simulink model "Biomasa_modelling"  (R2018a)
settings: Solver=ode23  StartTime=0.0  StopTime=120  RelTol=1e-3
InitFcn:
  | parametros_BIO
values from neighbouring files (symbols this model uses):
  b = 4.91    [SimulinkInit.m]    (also in parametros_BIO.m)
  C = 1    [SimulinkInit.m]    (also in parametros_BIO.m)
  K = 25    [SimulinkInit.m]    (also in parametros_BIO.m; uio_linear.m = K1+E*H)
  K1 = 9.66    [SimulinkInit.m]    (also in parametros_BIO.m; uio_linear.m = K1')
  K11 = 0.8    [SimulinkInit.m]    (also in parametros_BIO.m)
  K2 = 6.97    [SimulinkInit.m]    (also in parametros_BIO.m)
  K22 = 0.2    [SimulinkInit.m]    (also in parametros_BIO.m)
  K3 = 31.8    [SimulinkInit.m]    (also in parametros_BIO.m)
  K33 = 0.23    [SimulinkInit.m]    (also in parametros_BIO.m)
  K4 = 15.1    [SimulinkInit.m]    (also in parametros_BIO.m)
  Kd = 0.02    [SimulinkInit.m]    (also in parametros_BIO.m)
  Kdc = 0.02    [SimulinkInit.m]    (also in parametros_BIO.m)
  Kf = 1    [SimulinkInit.m]    (also in parametros_BIO.m)
  Kh = 1.2    [SimulinkInit.m]    (also in parametros_BIO.m)
  Ks = 21.5    [SimulinkInit.m]    (also in parametros_BIO.m)
  Ksc = 3    [SimulinkInit.m]    (also in parametros_BIO.m)
  Kv = 1    [SimulinkInit.m]    (also in parametros_BIO.m)
  Sbin = 13.8    [SimulinkInit.m]    (also in parametros_BIO.m)
  Svin = 2.91    [SimulinkInit.m]    (also in parametros_BIO.m)
  T1 = 0.4    [SimulinkInit.m]    (also in parametros_BIO.m)
  T2 = 1    [SimulinkInit.m]    (also in parametros_BIO.m)
  T3 = 15    [SimulinkInit.m]    (also in parametros_BIO.m)
  T4 = 2.5    [SimulinkInit.m]    (also in parametros_BIO.m)
  T5 = 3.3    [SimulinkInit.m]    (also in parametros_BIO.m)
  Tcd = 0.2    [SimulinkInit.m]    (also in parametros_BIO.m)
  Tcr = 0.01    [SimulinkInit.m]    (also in parametros_BIO.m)
  Tf = 0.04    [SimulinkInit.m]    (also in parametros_BIO.m)
  Tr = 950    [SimulinkInit.m]    (also in parametros_BIO.m)
  Tt = 450    [SimulinkInit.m]    (also in parametros_BIO.m)
  Ttd = 0.04    [SimulinkInit.m]    (also in parametros_BIO.m)
  Tv = 0.05    [SimulinkInit.m]    (also in parametros_BIO.m)
  V = 20    [SimulinkInit.m]    (also in parametros_BIO.m)
  wref = 70000    [SimulinkInit.m]    (also in parametros_BIO.m)
  X_acid = 1.2    [SimulinkInit.m]    (also in parametros_BIO.m)
  X_meth = 0.35    [SimulinkInit.m]    (also in parametros_BIO.m)
  Z = 3    [SimulinkInit.m]    (also in parametros_BIO.m)
libraries: powerlib x3
settings Model: Creator=cmparedes  LastModifiedBy=cmparedes
settings SolverCC: AlgebraicLoopSolver=LineSearch

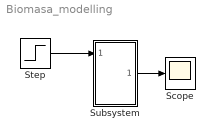
== system Biomasa_modelling ==
  Scope : Scope
  Step : Step  Time=0  After=28  SampleTime=0
  Subsystem : Subsystem
  wires:
  Step/1 -> Subsystem/1(In1)
  Subsystem/1(Vdc) -> Scope/1

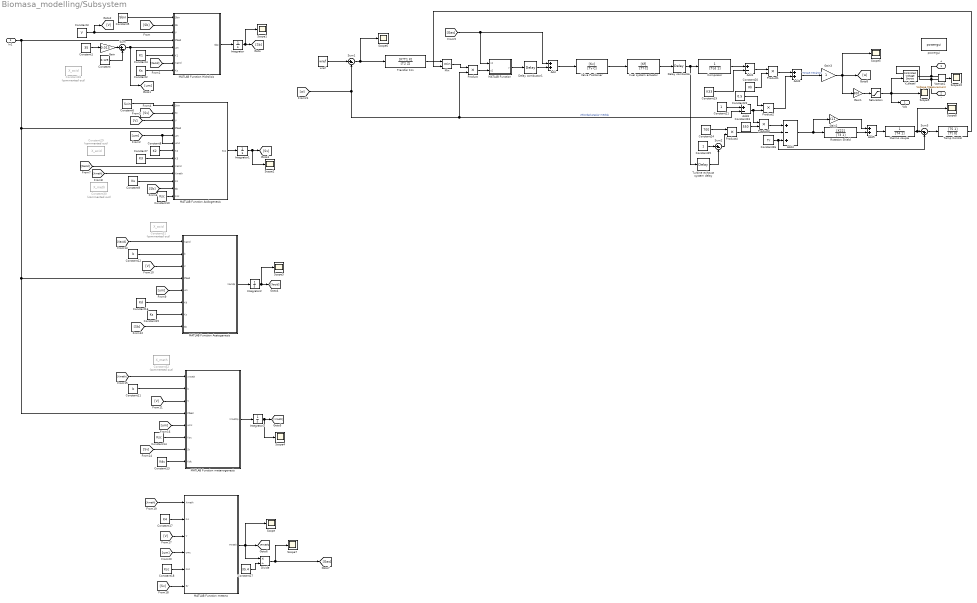
== system Biomasa_modelling/Subsystem ==
  In1 : Inport
  Add : Sum
  Add1 : Sum  Inputs=+-
  Add2 : Sum
  Add3 : Sum  Inputs=+-
  Add4 : Sum  Inputs=+-+
  Add5 : Sum
  Compresor : TransferFcn  Denominator=[Tcd 1]
  Constant : Constant  Value=0.129
  Constant1 : Constant  Value=35
  Constant10 : Constant  Value=Ksc
  Constant11 : Constant  Value=b
  Constant12 : Constant  Value=b
  Constant13 : Constant  Value=Kdc
  Constant14 : Constant  Value=Ksc
  Constant15 : Constant  Value=Ks
  Constant16 : Constant  Value=Kd
  Constant17 : Constant  Value=K4
  Constant18 : Constant  Value=Ksc
  Constant19 : Constant  Value=K33
  Constant2 : Constant  Value=Ks
  Constant20 : Constant  Value=Kh
  Constant21 : Constant
  Constant22 : Constant  Value=0.5
  Constant23 : Constant  Value=550
  Constant24 : Constant  Value=700
  Constant25 : Constant
  Constant26 : Constant  Value=Tr
  Constant27 : Constant  Value=35.4
  Constant28 : Constant  Commented=on  Value=X_acid
  Constant29 : Constant  Commented=on  Value=X_acid
  Constant3 : Constant  Value=V
  Constant30 : Constant  Commented=on  Value=X_meth
  Constant31 : Constant  Commented=on  Value=X_acid
  Constant32 : Constant  Commented=on  Value=X_meth
  Constant4 : Constant  Value=K1
  Constant5 : Constant  Value=Sbin
  Constant6 : Constant  Value=Svin
  Constant7 : Constant  Value=K3
  Constant8 : Constant  Value=K2
  Constant9 : Constant  Value=Ks
  Delay combustor : TransportDelay  DelayTime=Tcr
  Delay combustor1 : TransportDelay  DelayTime=0
  Divide : Product  Inputs=*/
  Fuel system actuator : TransferFcn  Numerator=[Kf]  Denominator=[Tf C]
  Gain : Gain  Gain=0.013
  Gain1 : Gain  Gain=900
  Gain2 : Gain  Gain=K11
  Gain3 : Gain
  Integrator : Integrator
  Integrator1 : Integrator
  Integrator2 : Integrator  InitialCondition=1.2
  Integrator3 : Integrator  InitialCondition=0.35
  MATLAB Function : MATLAB Function  TreatAsAtomicUnit=on
  MATLAB Function Acetogenesis : MATLAB Function  TreatAsAtomicUnit=on
  MATLAB Function Acidogenesis : MATLAB Function  TreatAsAtomicUnit=on
  MATLAB Function Hidrolisis : MATLAB Function  TreatAsAtomicUnit=on
  MATLAB Function metano : MATLAB Function  TreatAsAtomicUnit=on
  MATLAB Function metanogenesis : MATLAB Function  TreatAsAtomicUnit=on
  Min : MinMax  Inputs=2
  Product{,1..4} (5 alike) : Product
  Rotation Shield : TransferFcn  Numerator=[K22]  Denominator=[T3 1]
  Saturation : Saturate  UpperLimit=1000  LowerLimit=0
  Scope{,1..10} (11 alike) : Scope
  Sum : Sum  Inputs=|+-
  Sum1 : Sum  Inputs=|+-
  Sum2 : Sum  Inputs=|+-
  Sum3 : Sum  Inputs=|-+
  Temp Control : TransferFcn  Numerator=[T5 1]  Denominator=[Tt 0]
  Transfer Fcn : TransferFcn  Numerator=[K*T1 K]  Denominator=[T2 Z]
  Turbine exhaust system delay : TransportDelay  DelayTime=Ttd
  V_diesel : powerlib/Electrical Sources/Controlled Voltage Source  Initialize=on  Source_Type=DC  Amplitude=0  Phase=0  Frequency=0  Measurements=None
  Valve Positioner : TransferFcn  Numerator=[Kv]  Denominator=[Tv C]
  Vsensa1 : powerlib/Measurements/Voltage Measurement  PhasorSimulation=off  OutputType=Complex  PSBequivalent=0
  powergui : powerlib/powergui  Priority=1  SimulationMode=Continuous  SampleTime=50e-6  frequency=60  Iterations=50  frequencyindice=0  Pbase=100e6  ErrMax=1e-4  UnitsV=kV  UnitsW=MW  buscounter=0  FunctionMessages=off  echomessages=off  EnableUseOfTLC=off  CurrentSourceSwitches=off  DisableSnubberDevices=off  DisableRonSwitches=off  DisableVfSwitches=off  DisplayEquations=off  SolverType=Tustin/Backward Euler (TBE)  Interpol=off  ExternalGateDelay=off  methode=off  Ts=100  x0status=blocks  SPID=on  SwTol=0  HookPort=off  RestoreLinks=warning  ResistiveCurrentMeasurement=off  Frange=[0:2:500]  Ylog=off  Xlog=on  ShowGrid=off  save=off  variable=ZData  structure=0  ZoomFFT=off  StartTime=0.0  cycles=1  DisplayStyle=1  fundamental=60  FreqAxis=off  MaxFrequency=1000  frequencyindicesteady=1  RmsSteady=1  display=off
  thermo couple : TransferFcn  Denominator=[T4 1]
  wref : Constant  Value=wref
  + : PMIOPort  Side=Left
  - : PMIOPort  Port=2  Side=Left
  Vdc : Outport
  wires:
  MATLAB Function metano/1(Fmeth) -> Divide/1, Scope/1, [Fmeth]
  Sum/1 -> [um], MATLAB Function Hidrolisis/5(um)
  Constant16/1 -> MATLAB Function Acetogenesis/6(Kd)
  Temp Control/1 -> Min/2
  Integrator/1 -> Scope1/1, [Sb]
  Gain3/1 -> Gain1/1, Scope5/1, [w]
  Sum1/1 -> Transfer Fcn/1, Scope6/1
  [Sb] -> MATLAB Function Acetogenesis/8(Sb)
  [Sv] -> MATLAB Function metanogenesis/7(Sv)
  Add4/1 -> Rotation Shield/1, Gain2/1
  Constant8/1 -> MATLAB Function Acidogenesis/7(K2)
  Constant24/1 -> Product4/1
  [V] -> MATLAB Function Acetogenesis/3(V)
  Constant23/1 -> Product3/2
  Constant27/1 -> Divide/2
  [Sb] -> MATLAB Function Acidogenesis/12(Sb)
  Integrator3/1 -> Scope4/1, [Xmeth]
  Integrator2/1 -> Scope3/1, [Xacid]
  Divide/1 -> Scope7/1, [Gas]
  Constant7/1 -> MATLAB Function Acidogenesis/8(K3)
  Delay combustor/1 -> Turbine exhaust system delay/1, Compresor/1
  [V] -> MATLAB Function Acidogenesis/3(V)
  Constant12/1 -> MATLAB Function Acetogenesis/2(b)
  Sum2/1 -> Product4/2
  [V] -> MATLAB Function metanogenesis/3(V)
  Gain/1 -> Sum/1
  Product/1 -> MATLAB Function/2(u2)
  [w] -> Product/2, Add3/2, Sum1/2  "velocidad angular medida"
  Constant6/1 -> MATLAB Function Acidogenesis/1(Svin)
  wref/1 -> Sum1/1
  [Gas] -> MATLAB Function/1(u1), Add/1
  [Sv] -> MATLAB Function metano/6(Sv)
  MATLAB Function Hidrolisis/1(Sbp) -> Integrator/1
  Turbine exhaust system delay/1 -> Sum2/2
  MATLAB Function Acetogenesis/1(Xacidp) -> Integrator2/1
  Constant/1 -> Sum/2
  Constant18/1 -> MATLAB Function metano/5(Ksc)
  In1/1 -> MATLAB Function Acidogenesis/4(Ffeed), MATLAB Function metanogenesis/4(Ffeed), MATLAB Function Acetogenesis/4(Ffeed), MATLAB Function Hidrolisis/4(Ffeed)
  Add3/1 -> Product3/1, Product2/2
  [um] -> MATLAB Function Acetogenesis/5(um)
  Product3/1 -> Add4/1
  Constant15/1 -> MATLAB Function Acetogenesis/7(Ks)
  thermo couple/1 -> Scope8/1, Sum3/1
  Fuel system actuator/1 -> Delay combustor/1
  Add/1 -> Valve Positioner/1
  Add5/1 -> thermo couple/1
  Gain2/1 -> Add5/1
  Constant22/1 -> Product2/1
  [um] -> MATLAB Function metano/4(umc)
  Compresor/1 -> Add1/1
  Constant10/1 -> MATLAB Function Acidogenesis/13(Ksc)
  [um] -> MATLAB Function Acidogenesis/6(umc), MATLAB Function Acidogenesis/5(um)
  Constant9/1 -> MATLAB Function Acidogenesis/11(Ks)
  Constant1/1 -> Gain/1
  Constant13/1 -> MATLAB Function metanogenesis/8(Kdc)
  Constant26/1 -> Sum3/2, Add4/3
  Integrator1/1 -> Scope2/1, [Sv]
  [Xmeth] -> MATLAB Function metanogenesis/1(Xmeth)
  Add2/1 -> Gain3/1  "Torque mecánico"
  MATLAB Function/1(y) -> Delay combustor1/1
  Saturation/1 -> Vdc/1, V_diesel/1, Scope9/1
  [Sb] -> MATLAB Function Hidrolisis/2(Sb)
  Min/1 -> Product/1
  Constant3/1 -> [V], MATLAB Function Hidrolisis/3(V)
  MATLAB Function Acidogenesis/1(Svp) -> Integrator1/1
  Constant5/1 -> MATLAB Function Hidrolisis/1(Sbin)
  Constant20/1 -> Product1/2
  [Xmeth] -> MATLAB Function Acidogenesis/10(Xmeth)
  Sum3/1 -> Temp Control/1
  Gain1/1 -> Saturation/1
  Constant21/1 -> Add3/1
  Constant25/1 -> Sum2/1
  Product2/1 -> Add2/2
  [Xacid] -> MATLAB Function Acidogenesis/9(Xacid)
  Valve Positioner/1 -> Fuel system actuator/1
  Constant4/1 -> MATLAB Function Hidrolisis/6(K1)
  Constant11/1 -> MATLAB Function metanogenesis/2(b)
  Rotation Shield/1 -> Add5/2
  Add1/1 -> Product1/1
  [Sv] -> MATLAB Function Acidogenesis/2(Sv)
  [Xacid] -> MATLAB Function Acetogenesis/1(Xacid)
  Constant19/1 -> Add1/2
  Product1/1 -> Add2/1
  Transfer Fcn/1 -> Min/1
  Delay combustor1/1 -> Add/2
  [um] -> MATLAB Function metanogenesis/5(umc)
  MATLAB Function metanogenesis/1(Xmethp) -> Integrator3/1
  Constant14/1 -> MATLAB Function metanogenesis/6(Ksc)
  Product4/1 -> Add4/2
  Constant2/1 -> MATLAB Function Hidrolisis/8(Ks)
  Constant17/1 -> MATLAB Function metano/2(K4)
  [V] -> MATLAB Function metano/3(V)
  [Xmeth] -> MATLAB Function metano/1(Xmeth)
  [Xacid] -> MATLAB Function Hidrolisis/7(Xacid)
  Vsensa1/1 -> Scope10/1
  connections:
  Vsensa1/LConn1 -- +/RConn1 -- V_diesel/RConn1
  Vsensa1/LConn2 -- -/RConn1 -- V_diesel/LConn1

== matlab function Biomasa_modelling/Subsystem/MATLAB Function Acidogenesis ==
  data: Svin input; Sv input; V input; Ffeed input; um input; umc input; K2 input; K3 input; Xacid input; Xmeth input; Ks input; Svp output; Sb input; Ksc input
function Svp = fcn(Svin,Sv,V,Ffeed,um,umc,K2,K3,Xacid,Xmeth,Ks,Sb,Ksc)

% Svp=(Svin-Sv)*(Ffeed/V)+um*K2*Xacid/(1+Ks/Sb)-umc*K3*Xmeth/(1+Ksc/Sv);
Svp=(Svin-Sv)*(Ffeed/V)+um*K2*Xacid/(Ks/(1+Sb))-umc*K3*Xmeth/(Ksc/(1+Sv));

== matlab function Biomasa_modelling/Subsystem/MATLAB Function Hidrolisis ==
  data: Sbin input; Sbp output; Sb input; V input; Ffeed input; um input; K1 input; Xacid input; Ks input
function Sbp = fcn(Sbin,Sb,V,Ffeed,um,K1,Xacid,Ks)

% Sbp=(Sbin-Sb)*(Ffeed/V)+um*K1*Xacid/(1+Ks/Sb);
Sbp=(Sbin-Sb)*(Ffeed/V)+um*K1*Xacid/(Ks/(1+Sb));

== matlab function Biomasa_modelling/Subsystem/MATLAB Function Acetogenesis ==
  data: Xacid input; b input; V input; Ffeed input; um input; Kd input; Ks input; Xacidp output; Sb input
function Xacidp = fcn(Xacid,b,V,Ffeed,um,Kd,Ks,Sb)

% Xacidp=(um/(1+Ks/Sb)-Kd-Ffeed/(b*V))*Xacid;
Xacidp=(um/(Ks/(1+Sb))-Kd-Ffeed/(b*V))*Xacid;

== matlab function Biomasa_modelling/Subsystem/MATLAB Function metanogenesis ==
  data: Xmeth input; b input; V input; Ffeed input; umc input; Ksc input; Sv input; Xmethp output; Kdc input
function Xmethp = fcn(Xmeth,b,V,Ffeed,umc,Ksc,Sv,Kdc)

% Xmethp=(umc/(Ksc/Sv+1)-Kdc-Ffeed/(b*V))*Xmeth;
Xmethp=(umc/(Ksc/(Sv+1))-Kdc-Ffeed/(b*V))*Xmeth;

== matlab function Biomasa_modelling/Subsystem/MATLAB Function metano ==
  data: Xmeth input; K4 input; V input; umc input; Ksc input; Sv input; Fmeth output
function Fmeth = fcn(Xmeth,K4,V,umc,Ksc,Sv)


% Fmeth=V*umc*K4*Xmeth/(Ksc/Sv+1);
Fmeth=V*umc*K4*Xmeth/(Ksc/(Sv+1));

== matlab function Biomasa_modelling/Subsystem/MATLAB Function ==
  data: u1 input; y output; u2 input
function y = fcn(u1,u2)

y = u2*(1-u1);
